simulink model "SupervisorFSM_TX"  (R2023b)
settings: configuration reference "AMCBLDC_Configuration" (kept outside this file)
libraries: simulink x2
settings Model: DataDictionary=amcbldc.sldd  Creator=vvasco  LastModifiedBy=mfussi
settings ConfigSetRef: SourceName=AMCBLDC_Configuration

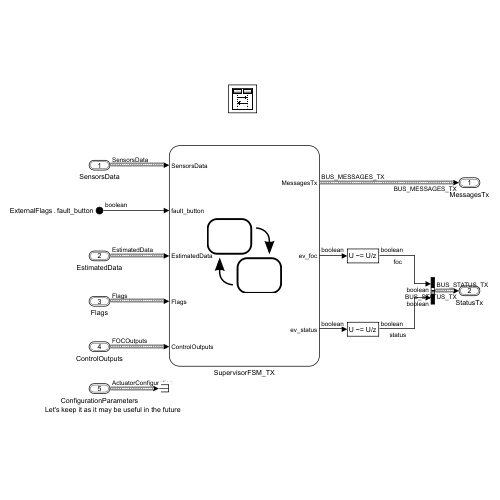
[thumbnail: Simulink's stored preview of the top-level diagram]
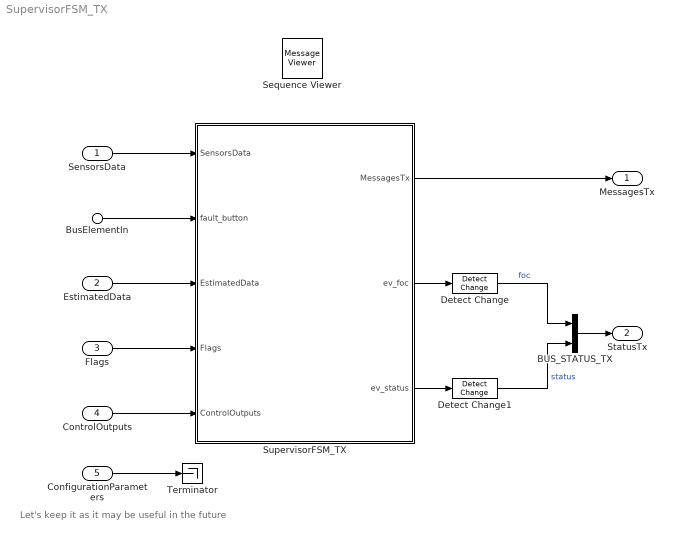
== system SupervisorFSM_TX ==
  note: Let's keep it as it may be useful in the future
  SensorsData : Inport  OutDataTypeStr=Bus: SensorsData  BusOutputAsStruct=on
  EstimatedData : Inport  Port=2  OutDataTypeStr=Bus: EstimatedData  BusOutputAsStruct=on
  Flags : Inport  Port=3  OutDataTypeStr=Bus: Flags  BusOutputAsStruct=on
  ControlOutputs : Inport  Port=4  OutDataTypeStr=Bus: FOCOutputs  BusOutputAsStruct=on
  ConfigurationParameters : Inport  Port=5  OutDataTypeStr=Bus: ActuatorConfiguration  BusOutputAsStruct=on
  BusElementIn : Inport  Port=6  PortName=ExternalFlags  Element=fault_button
  BUS_STATUS_TX : BusCreator  Inputs=2  OutDataTypeStr=Bus: BUS_STATUS_TX  NonVirtualBus=on
      settings: InheritFromInputs=off
  Detect Change : simulink/Logic and Bit Operations/Detect Change  vinit=false  OutDataTypeStr=boolean
  Detect Change1 : simulink/Logic and Bit Operations/Detect Change  vinit=false  OutDataTypeStr=boolean
  Sequence Viewer : MessageViewer  History=1000  SavedRootId=#
  SupervisorFSM_TX : Stateflow chart  TreatAsAtomicUnit=on
  Terminator : Terminator
  MessagesTx : Outport  OutDataTypeStr=Bus: BUS_MESSAGES_TX  BusOutputAsStruct=on
  StatusTx : Outport  Port=2  OutDataTypeStr=Bus: BUS_STATUS_TX  BusOutputAsStruct=on
  wires:
  SupervisorFSM_TX/1(MessagesTx) -> MessagesTx/1
  SensorsData/1 -> SupervisorFSM_TX/1(SensorsData)
  Flags/1 -> SupervisorFSM_TX/4(Flags)
  BUS_STATUS_TX/1 -> StatusTx/1
  EstimatedData/1 -> SupervisorFSM_TX/3(EstimatedData)
  ControlOutputs/1 -> SupervisorFSM_TX/5(ControlOutputs)
  SupervisorFSM_TX/2(ev_foc) -> Detect Change/1
  Detect Change/1 -> BUS_STATUS_TX/1  "foc"
  SupervisorFSM_TX/3(ev_status) -> Detect Change1/1
  Detect Change1/1 -> BUS_STATUS_TX/2  "status"
  ConfigurationParameters/1 -> Terminator/1
  BusElementIn/1 -> SupervisorFSM_TX/2(fault_button)

== stateflow chart SupervisorFSM_TX/SupervisorFSM_TX ==
  state MSG_FOC_HANDLER [parallel]
    settings: executionOrder=1
    state Home
    (default) -> MSG_FOC_HANDLER.Home
    MSG_FOC_HANDLER.Home -> MSG_FOC_HANDLER.Home : [Flags.enable_sending_msg_status]
        | {MessagesTx.foc.current = EstimatedData.Iq_filtered;
        | MessagesTx.foc.velocity = EstimatedData.velocity;
        | MessagesTx.foc.position = SensorsData.position;
        | send(ev_foc);}
  state MSG_STATUS_HANDLER [parallel]
    settings: executionOrder=2
    state Home
    (default) -> MSG_STATUS_HANDLER.Home
    MSG_STATUS_HANDLER.Home -> MSG_STATUS_HANDLER.Home : [Flags.enable_sending_msg_status]
        | {MessagesTx.status.control_mode = convert(Flags.control_mode);
        | MessagesTx.status.pwm_fbk = ControlOutputs.Vq;
        | MessagesTx.status.flags.ExternalFaultAsserted = fault_button;
        | MessagesTx.status.flags.OverCurrentFailure = Flags.hw_faults.overcurrent;
        | send(ev_status);}
  data: mccontrolmode function_output Enum: MCControlModes size=1; controlmode function_input Enum: ControlModes size=1; MessagesTx output Bus: BUS_MESSAGES_TX; SensorsData input Bus: SensorsData; fault_button input; EstimatedData input Bus: EstimatedData; Flags input Bus: Flags; ControlOutputs input Bus: FOCOutputs
  events: ev_foc output EITHER_EDGE_EVENT; ev_status output EITHER_EDGE_EVENT
  function mccontrolmode = convert(controlmode):
    | function mccontrolmode = convert(controlmode)
    | 
    | if controlmode == ControlModes.Idle
    |     mccontrolmode = MCControlModes.Idle;
    | elseif controlmode == ControlModes.Current
    |     mccontrolmode = MCControlModes.Current;
    | elseif controlmode == ControlModes.Velocity
    |     mccontrolmode = MCControlModes.SpeedVoltage;
    | elseif controlmode == ControlModes.Voltage
    |     mccontrolmode = MCControlModes.OpenLoop;
    | elseif controlmode == ControlModes.HwFaultCM
    |     mccontrolmode = MCControlModes.HWFault;
    | else
    |     mccontrolmode = MCControlModes.Idle;
    | end
    | 
    | end
